simulink model "DalinovRegulator"  (R2013b)
settings: Solver=ode45  StartTime=0.0  StopTime=10.0  RelTol=1e-3
settings Model: Creator=Darko  LastModifiedBy=Darko
settings DebuggingCC: SolverPrmCheckMsg=none

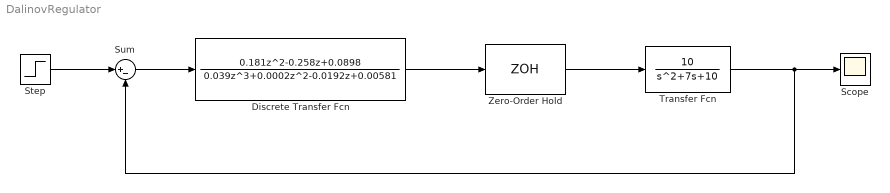
== system DalinovRegulator ==
  Discrete Transfer Fcn : DiscreteTransferFcn  Numerator=[0.181 -0.258 0.0898]  Denominator=[0.039 0.0002 -0.0192 0.00581]  SampleTime=0.1
  Scope : Scope
  Step : Step  Time=0  SampleTime=0.01
  Sum : Sum  Inputs=|+-
  Transfer Fcn : TransferFcn  Numerator=[10]  Denominator=[1 7 10]
  Zero-Order Hold : ZeroOrderHold  SampleTime=0.1
  wires:
  Step/1 -> Sum/1
  Sum/1 -> Discrete Transfer Fcn/1
  Discrete Transfer Fcn/1 -> Zero-Order Hold/1
  Zero-Order Hold/1 -> Transfer Fcn/1
  Transfer Fcn/1 -> Sum/2, Scope/1
